simulink model "aquabot_main"  (R2023b)
settings: Solver=FixedStepAuto  StartTime=0.0  StopTime=Inf  RelTol=1e-3
model workspace (MAT data in the model file):
  SL_Bus_ROSEnable64bitIntegers = 1
  SL_ROS_VariableLengthArrays_MaxSizes.CommonInfo.ArrayTruncateAction = 'EmitWarning'
  SL_ROS_VariableLengthArrays_MaxSizes.MsgTypeMap = containers.Map
  SL_ROS_VariableLengthArrays_MaxSizes.MsgTypeMap.serialization.keys = {'nav_msgs/OccupancyGrid', 'sensor_msgs/LaserScan'}
  SL_ROS_VariableLengthArrays_MaxSizes.MsgTypeMap.serialization.values{1}.PropertyName = 'data'
  SL_ROS_VariableLengthArrays_MaxSizes.MsgTypeMap.serialization.values{1}.DataType = 'int8'
  SL_ROS_VariableLengthArrays_MaxSizes.MsgTypeMap.serialization.values{1}.MaxLength = 422500
  SL_ROS_VariableLengthArrays_MaxSizes.MsgTypeMap.serialization.values{2}(1).PropertyName = 'intensities'
  SL_ROS_VariableLengthArrays_MaxSizes.MsgTypeMap.serialization.values{2}(1).DataType = 'single'
  SL_ROS_VariableLengthArrays_MaxSizes.MsgTypeMap.serialization.values{2}(1).MaxLength = 1875
  SL_ROS_VariableLengthArrays_MaxSizes.MsgTypeMap.serialization.values{2}(2).PropertyName = 'ranges'
  SL_ROS_VariableLengthArrays_MaxSizes.MsgTypeMap.serialization.values{2}(2).DataType = 'single'
  SL_ROS_VariableLengthArrays_MaxSizes.MsgTypeMap.serialization.values{2}(2).MaxLength = 1875
  SL_ROS_VariableLengthArrays_MaxSizes.MsgTypeMap.serialization.uniformity = 0
  SL_ROS_VariableLengthArrays_MaxSizes.MsgTypeMap.serialization.keyType = 'char'
  SL_ROS_VariableLengthArrays_MaxSizes.MsgTypeMap.serialization.valueType = 'any'
libraries: ros2lib x8
settings Model: Creator=nicolas  LastModifiedBy=nicolas
settings OptimizationCC: EnhancedBackFolding=on  PassReuseOutputArgsAs=Individual arguments  ZeroExternalMemoryAtStartup=off  ZeroInternalMemoryAtStartup=off  MaxStackSize=64  OptimizeBlockOrder=speed  DifferentSizesBufferReuse=on  OptimizationCustomize=off  EfficientTunableParamExpr=on
settings DebuggingCC: ParameterTunabilityLossMsg=error
settings HardwareCC: ProdBitPerLong=64  ProdHWDeviceType=Intel->x86-64 (Linux 64)  UseEmbeddedCoderFeatures=off
settings RTWCC: Description=Embedded Coder  SystemTargetFile=ert.tlc  HardwareBoard=Robot Operating System 2 (ROS 2)  TLCOptions="-aInlineSetEventsForThisBaseRateFcn=TLC_FALSE -aSuppressMultiTaskScheduler=TLC_FALSE  -aRateBasedStepFcn=0"  TemplateMakefile=ert_default_tmf  Toolchain=Colcon Tools  TargetLang=C++
settings CodeAppCC: ForceParamTrailComments=on  IgnoreCustomStorageClasses=off  OperatorAnnotations=on  SimulinkDataObjDesc=on  SFDataObjDesc=on  InsertBlockDesc=on
settings ERTTargetCC: CodeInterfacePackaging=C++ class  SupportNonInlinedSFcns=on  RootIOFormat=Structure reference

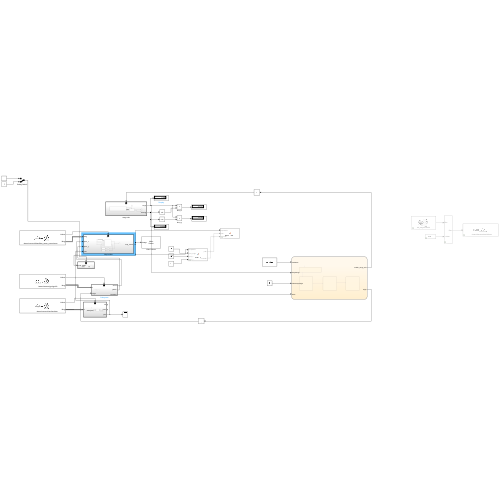
[thumbnail: Simulink's stored preview of the top-level diagram]
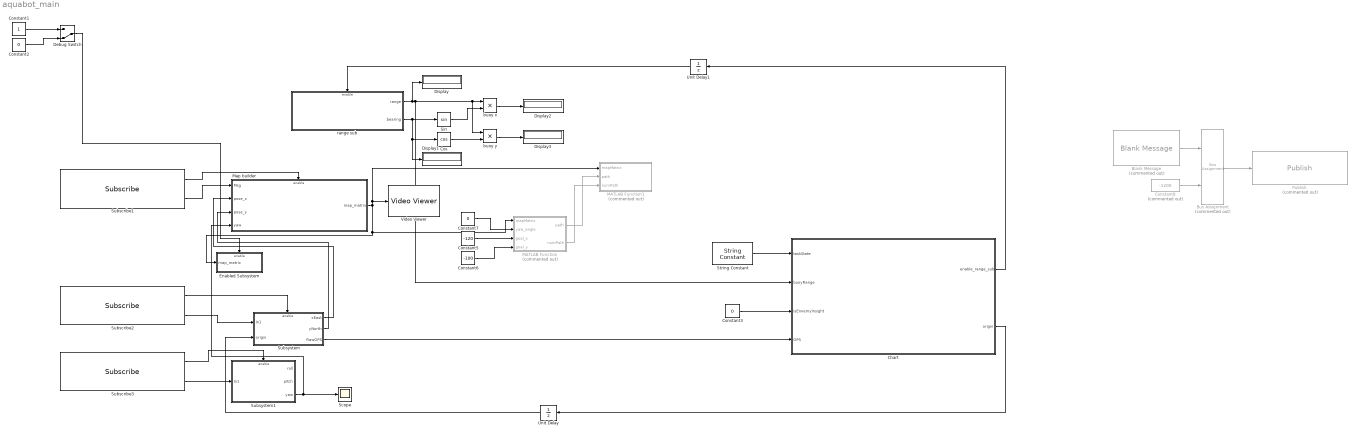
== system aquabot_main ==
  Blank Message : ros2lib/Blank Message  Commented=on  messageClass=Message  entityType=std_msgs/Float64  messageType=std_msgs/Float64  SampleTime=inf
  Bus Assignment : BusAssignment  Commented=on  AssignedSignals=data
  Chart : Stateflow chart  TreatAsAtomicUnit=on
  Constant1 : Constant
  Constant2 : Constant  Value=0
  Constant3 : Constant  Value=0
  Constant5 : Constant  Value=-120
  Constant6 : Constant  Value=-100
  Constant7 : Constant  Value=0
  Constant8 : Constant  Commented=on  Value=-1200
  Cos : Trigonometry  Operator=cos
  Debug Switch : ManualSwitch  CurrentSetting=0
  Display{,1..3} (4 alike) : Display
  Enabled Subsystem : Subsystem  TreatAsAtomicUnit=on
  MATLAB Function : MATLAB Function  Commented=on  TreatAsAtomicUnit=on
  MATLAB Function1 : MATLAB Function  Commented=on  TreatAsAtomicUnit=on
  Map builder : Subsystem
  Publish : ros2lib/Publish  Commented=on  topicSource=Select from ROS network  topic=/wamv/thrusters/main/thrust  messageType=std_msgs/Float64  QOSHistory=Keep last  QOSDepth=1  QOSReliability=Reliable  QOSDurability=Volatile
  Scope : Scope
  Sin : Trigonometry
  String Constant : StringConstant  String="\"running\""
  Subscribe1 : ros2lib/Subscribe  topicSource=Select from ROS network  topic=/wamv/sensors/lidars/lidar_wamv_sensor/scan  messageType=sensor_msgs/LaserScan  sampleTime=-1  QOSHistory=Keep last  QOSDepth=1  QOSReliability=Reliable  QOSDurability=Volatile
  Subscribe2 : ros2lib/Subscribe  topicSource=Select from ROS network  topic=/wamv/sensors/gps/gps/fix  messageType=sensor_msgs/NavSatFix  sampleTime=-1  QOSHistory=Keep last  QOSDepth=1  QOSReliability=Reliable  QOSDurability=Volatile
  Subscribe3 : ros2lib/Subscribe  topicSource=Select from ROS network  topic=/wamv/sensors/imu/imu/data  messageType=sensor_msgs/Imu  sampleTime=-1  QOSHistory=Keep last  QOSDepth=1  QOSReliability=Reliable  QOSDurability=Volatile
  Subsystem : Subsystem
  Subsystem1 : Subsystem
  Unit Delay : UnitDelay  InitialCondition=[0 0]  SampleTime=-1  HasFrameUpgradeWarning=on
  Unit Delay1 : UnitDelay  SampleTime=-1  HasFrameUpgradeWarning=on
  Video Viewer : VideoViewer  FigPos=[681 999 1074 725]
  buoy x : Product
  buoy y : Product
  range sub : Subsystem
  wires:
  Subscribe1/2 -> Map builder/1(Msg)
  Subscribe1/1 -> Map builder/Enable
  Subscribe3/2 -> Subsystem1/1(In1)
  Subscribe3/1 -> Subsystem1/Enable
  Constant1/1 -> Debug Switch/1
  Constant2/1 -> Debug Switch/2
  Map builder/1(map_matrix) -> Video Viewer/1, MATLAB Function1/1(mapMatrix), Enabled Subsystem/1(map_matrix), MATLAB Function/1(mapMatrix)
  Debug Switch/1 -> Enabled Subsystem/Enable
  Constant3/1 -> Chart/3(isEnnemyInsight)
  range sub/1(range) -> buoy x/1, buoy y/1, Chart/2(buoyRange), Display/1
  String Constant/1 -> Chart/1(taskState)
  Subsystem1/3(yaw) -> Map builder/4(yaw), Scope/1
  range sub/2(bearing) -> Sin/1, Cos/1, Display1/1
  Chart/1(enable_range_sub) -> Unit Delay1/1
  Sin/1 -> buoy x/2
  Cos/1 -> buoy y/2
  buoy x/1 -> Display2/1
  buoy y/1 -> Display3/1
  MATLAB Function/1(path) -> MATLAB Function1/2(path)
  MATLAB Function/2(numPath) -> MATLAB Function1/3(numPath)
  Constant5/1 -> MATLAB Function/3(goal_x)
  Constant6/1 -> MATLAB Function/4(goal_y)
  Constant7/1 -> MATLAB Function/2(yaw_angle)
  Blank Message/1 -> Bus Assignment/1
  Constant8/1 -> Bus Assignment/2
  Bus Assignment/1 -> Publish/1
  Subscribe2/2 -> Subsystem/1(In1)
  Chart/2(origin) -> Unit Delay/1
  Subsystem/3(RawGPS) -> Chart/4(GPS)
  Subscribe2/1 -> Subsystem/Enable
  Unit Delay/1 -> Subsystem/2(origin)
  Unit Delay1/1 -> range sub/Enable
  Subsystem/1(xEast) -> Map builder/2(pose_x)
  Subsystem/2(yNorth) -> Map builder/3(pose_y)

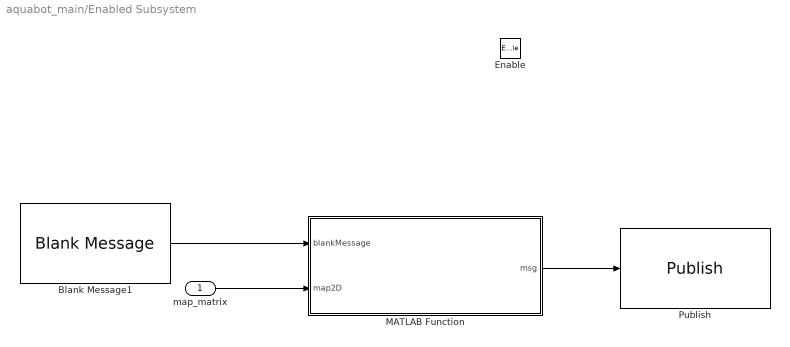
== system aquabot_main/Enabled Subsystem ==
  map_matrix : Inport
  Enable : EnablePort
  Blank Message1 : ros2lib/Blank Message  messageClass=Message  entityType=nav_msgs/OccupancyGrid  messageType=nav_msgs/OccupancyGrid  SampleTime=inf
  MATLAB Function : MATLAB Function  TreatAsAtomicUnit=on
  Publish : ros2lib/Publish  topicSource=Specify your own  topic=/siera/debug/map  messageType=nav_msgs/OccupancyGrid  QOSHistory=Keep last  QOSDepth=1  QOSReliability=Reliable  QOSDurability=Volatile
  wires:
  map_matrix/1 -> MATLAB Function/2(map2D)
  MATLAB Function/1(msg) -> Publish/1
  Blank Message1/1 -> MATLAB Function/1(blankMessage)

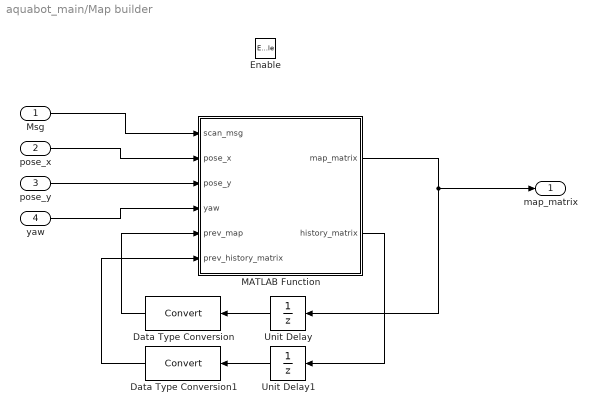
== system aquabot_main/Map builder ==
  Msg : Inport
  pose_x : Inport  Port=2
  pose_y : Inport  Port=3
  yaw : Inport  Port=4
  Enable : EnablePort
  Data Type Conversion : DataTypeConversion  SaturateOnIntegerOverflow=off  RndMeth=Floor
  Data Type Conversion1 : DataTypeConversion  SaturateOnIntegerOverflow=off  RndMeth=Floor
  MATLAB Function : MATLAB Function  TreatAsAtomicUnit=on
  Unit Delay : UnitDelay  InitialCondition=zeros(650,650,'logical')  SampleTime=-1  HasFrameUpgradeWarning=on
  Unit Delay1 : UnitDelay  InitialCondition=zeros(650,650,'uint8')  SampleTime=-1  HasFrameUpgradeWarning=on
  map_matrix : Outport
  wires:
  Msg/1 -> MATLAB Function/1(scan_msg)
  MATLAB Function/1(map_matrix) -> Unit Delay/1, map_matrix/1
  pose_x/1 -> MATLAB Function/2(pose_x)
  pose_y/1 -> MATLAB Function/3(pose_y)
  yaw/1 -> MATLAB Function/4(yaw)
  Unit Delay/1 -> Data Type Conversion/1
  Data Type Conversion/1 -> MATLAB Function/5(prev_map)
  MATLAB Function/2(history_matrix) -> Unit Delay1/1
  Data Type Conversion1/1 -> MATLAB Function/6(prev_history_matrix)
  Unit Delay1/1 -> Data Type Conversion1/1

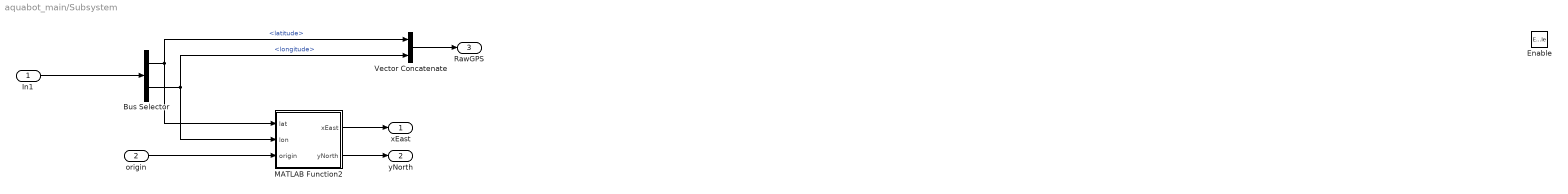
== system aquabot_main/Subsystem ==
  In1 : Inport
  origin : Inport  Port=2
  Enable : EnablePort
  Bus Selector : BusSelector  OutputSignals=latitude,longitude
  MATLAB Function2 : MATLAB Function  TreatAsAtomicUnit=on
  Vector Concatenate : Concatenate
  xEast : Outport
  yNorth : Outport  Port=2
  RawGPS : Outport  Port=3
  wires:
  In1/1 -> Bus Selector/1
  Bus Selector/1 -> MATLAB Function2/1(lat), Vector Concatenate/1  "<latitude>"
  Vector Concatenate/1 -> RawGPS/1
  Bus Selector/2 -> MATLAB Function2/2(lon), Vector Concatenate/2  "<longitude>"
  origin/1 -> MATLAB Function2/3(origin)
  MATLAB Function2/1(xEast) -> xEast/1
  MATLAB Function2/2(yNorth) -> yNorth/1

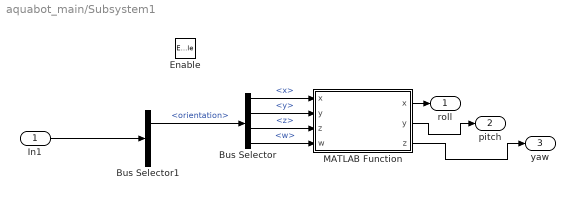
== system aquabot_main/Subsystem1 ==
  In1 : Inport
  Enable : EnablePort
  Bus Selector : BusSelector  OutputSignals=x,y,z,w
  Bus Selector1 : BusSelector  OutputSignals=orientation,angular_velocity
  MATLAB Function : MATLAB Function  TreatAsAtomicUnit=on
  roll : Outport
  pitch : Outport  Port=2
  yaw : Outport  Port=3
  wires:
  Bus Selector1/1 -> Bus Selector/1  "<orientation>"
  Bus Selector/2 -> MATLAB Function/2("y ")  "<y>"
  Bus Selector/4 -> MATLAB Function/4(w)  "<w>"
  Bus Selector/3 -> MATLAB Function/3("z ")  "<z>"
  MATLAB Function/2(y) -> pitch/1
  Bus Selector/1 -> MATLAB Function/1("x ")  "<x>"
  In1/1 -> Bus Selector1/1
  MATLAB Function/3(z) -> yaw/1
  MATLAB Function/1(x) -> roll/1

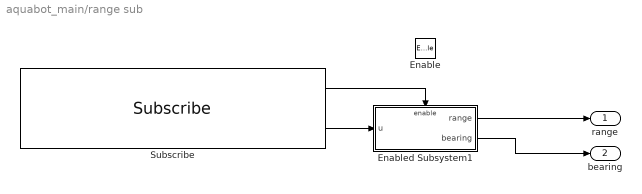
== system aquabot_main/range sub ==
  Enable : EnablePort
  Enabled Subsystem1 : Subsystem  TreatAsAtomicUnit=on
  Subscribe : ros2lib/Subscribe  topicSource=Select from ROS network  topic=/wamv/sensors/acoustics/receiver/range_bearing  messageType=ros_gz_interfaces/ParamVec  sampleTime=-1  QOSHistory=Keep last  QOSDepth=1  QOSReliability=Reliable  QOSDurability=Volatile
  range : Outport
  bearing : Outport  Port=2
  wires:
  Subscribe/1 -> Enabled Subsystem1/Enable
  Subscribe/2 -> Enabled Subsystem1/1(u)
  Enabled Subsystem1/2(bearing) -> bearing/1
  Enabled Subsystem1/1(range) -> range/1

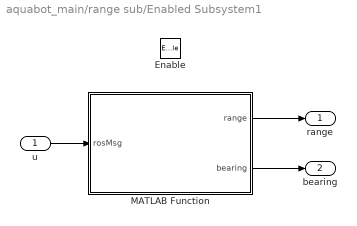
== system aquabot_main/range sub/Enabled Subsystem1 ==
  u : Inport
  Enable : EnablePort
  MATLAB Function : MATLAB Function  TreatAsAtomicUnit=on
  range : Outport
  bearing : Outport  Port=2
  wires:
  u/1 -> MATLAB Function/1(rosMsg)
  MATLAB Function/1(range) -> range/1
  MATLAB Function/2(bearing) -> bearing/1

== matlab function aquabot_main/Map builder/MATLAB Function ==
  data: scan_msg input; map_matrix output; pose_x input; pose_y input; yaw input; prev_map input; history_matrix output; prev_history_matrix input
function [map_matrix, history_matrix]= fcn(scan_msg, pose_x, pose_y, yaw, prev_map, prev_history_matrix)
    persistent num_iter;
    if isempty(num_iter)
        num_iter = 0;
    end

    ranges = scan_msg.ranges;
    ranges(ranges==inf) = NaN;
    angles = transpose(linspace(scan_msg.angle_min, scan_msg.angle_max, length(ranges)));
    % ox = ranges.*cos(angles);
    % oy = ranges.*sin(angles);
    % 
    % ox_corr = ox(isfinite(ox));
    % oy_corr = oy(isfinite(oy));

    map = binaryOccupancyMap(prev_map,1);
    map.GridOriginInLocal = -[diff(map.XWorldLimits) diff(map.YWorldLimits)]/2;
    insertRay(map, [pose_x pose_y yaw], ranges, angles, 130);
    map_matrix = map.occupancyMatrix();
    
    find_mm = find(map_matrix);
    prev_history_matrix(find_mm) = prev_history_matrix(find_mm) + 1;

    % if ~isempty(ox_corr)
    %     map.setOccupancy([ox_corr oy_corr], 1);
    % end
    % map_matrix = zeros(650, 650);
    num_iter = num_iter + 1;
end

== matlab function aquabot_main/Subsystem1/MATLAB Function ==
  data: x output; x input; y output; y input; z input; w input; z output
function [x, y, z]= quatToEuler(x, y, z, w)
    eulZYX = quat2eul([w, x, y, z], "ZYX");
    x = eulZYX(3);
    y = eulZYX(2);
    z = eulZYX(1);
end

== stateflow chart aquabot_main/Chart ==
  state Init
    entry:
  state SeekBuoy
    entry:
    origin = [GPS(1) GPS(2)]
    enable_range_sub=1;
  state Patroll
  state Follow
  (default) -> Init
  Init -> SeekBuoy : [taskState=="running" && all(GPS)~=0]
  Patroll -> Follow : [isEnnemyInsight==1]
  SeekBuoy -> Patroll : [buoyRange<=10]
  data: taskState input; buoyRange input; isEnnemyInsight input; enable_range_sub output; origin output; GPS input; worldmap local

== matlab function aquabot_main/Enabled Subsystem/MATLAB Function ==
  data: blankMessage input; map2D input; msg output Bus: SL_Bus_nav_msgs_OccupancyGrid
function msg = createOccupancyMsg(blankMessage, map2D)
    strFrameId = 'wamv/wamv/base_link';
    blankMessage.header.frame_id(1:length(strFrameId)) = uint8(strFrameId);
    blankMessage.header.frame_id_SL_Info.CurrentLength = uint32(length(strFrameId));
    blankMessage.info.resolution = single(1);
    blankMessage.info.width = uint32(size(map2D,1));
    blankMessage.info.height = uint32(size(map2D,2));
    blankMessage.info.origin.position.x = -130.0;
    blankMessage.info.origin.position.y = 130.0;
    blankMessage.info.origin.position.z = 0.0;
    blankMessage.info.origin.orientation.x = 0.0;
    blankMessage.info.origin.orientation.y = 0.0;
    blankMessage.info.origin.orientation.z = -0.707;
    blankMessage.info.origin.orientation.w = 0.707;
    map1D = map2D(:);
    blankMessage.data = int8(map1D).*100;
    blankMessage.data_SL_Info.CurrentLength = uint32(length(map1D));
    msg = blankMessage;
end

== matlab function aquabot_main/range sub/Enabled Subsystem1/MATLAB Function ==
  data: rosMsg input; range output; bearing output
function [range, bearing] = extractRangeFromParamVec(rosMsg)
    range = 0;
    bearing = 0;
    for param = rosMsg.params.'
        if param.value.type ~= 0
            if strncmp(char(param.name), 'range', param.name_SL_Info.CurrentLength)
                range = param.value.double_value;
            end
            if strncmp(char(param.name), 'bearing', param.name_SL_Info.CurrentLength)
                bearing = param.value.double_value;
            end
        end
    end
end

== matlab function aquabot_main/MATLAB Function ==
  data: mapMatrix input; path output; numPath output; yaw_angle input; goal_x input; goal_y input
function [path, numPath] = planner(mapMatrix, yaw_angle, goal_x, goal_y)
    MaxPathNum = 100;
    map = binaryOccupancyMap(mapMatrix, 1);
    map.GridOriginInLocal = [-130 -130];
    
    ss = stateSpaceSE2;
    ss.StateBounds = [map.XWorldLimits;map.YWorldLimits;[-pi pi]];

    sv = validatorOccupancyMap(ss,Map=map);


    planner = plannerHybridAStar(sv, MinTurningRadius=4, MotionPrimitiveLength=6, InterpolationDistance=4);
    startPose = [0 0 yaw_angle]; % [meters, meters, radians]
    goalPose = [goal_x goal_y atan2(goal_y, goal_x)];
    refpath = plan(planner,startPose,goalPose);
    path = zeros(MaxPathNum,3);
    path(1:refpath.NumStates,:) = refpath.States;
    numPath=refpath.NumStates;
end

== matlab function aquabot_main/MATLAB Function1 ==
  data: mapMatrix input; path input; numPath input
function viewDebug(mapMatrix, path, numPath)
    [r,c] = ind2sub(size(mapMatrix), find(mapMatrix));
    r = 130 - r;
    c = c - 130;
    
    hold off
    scatter(c,r,'filled','square','MarkerFaceColor','k')
    hold on
    scatter(path(2:numPath-1,1),path(2:numPath-1,2),'o','MarkerFaceColor','b')
    scatter(path(1,1),path(1,2),'o','MarkerFaceColor','g')
    scatter(path(numPath,1),path(numPath,2),'o','MarkerFaceColor','r')
    % for iPose = 1:numPath
        range = 10;
        quiver(path(1:numPath,1), path(1:numPath,2), range*cos(path(1:numPath,3)), range*sin(path(1:numPath,3)))
    % end
    xlim([-130 130])
    ylim([-130 130])
end

== matlab function aquabot_main/Subsystem/MATLAB Function2 ==
  data: xEast output; yNorth output; lat input; lon input; origin input
function [xEast,yNorth] = GPS2XY(lat,lon, origin)
    earth_radius = 6371000.0;
    
    if all(origin == 0)
        xEast = 0;
        yNorth = 0;
    else
        xEast = earth_radius * cos(deg2rad(lat - origin(1))) * sin(deg2rad(lon - origin(2)));
        yNorth = earth_radius * sin(deg2rad(lat - origin(1)));
    end
end
